simulink model "RailP_VD"  (R2018a)
settings: configuration reference "cs_ert" (kept outside this file)
values from neighbouring files (symbols this model uses):
  RailP_facFlt1PT1_C = 50.0    [RailP_VD.sldd]
  RailP_facFlt2PT1_C = 50.0    [RailP_VD.sldd]
  RailP_facFlt3PT1_C = 50.0    [RailP_VD.sldd]
  RailP_nDiffMax_C = 0.0    [RailP_VD.sldd]
  RailP_numMax_CUR : value not decoded    [RailP_VD.sldd]
  RailP_numMax_CURX : value not decoded    [RailP_VD.sldd]
  RailP_pFltWinNeg_CUR : value not decoded    [RailP_VD.sldd]
  RailP_pFltWinNeg_CURX : value not decoded    [RailP_VD.sldd]
  RailP_swtFlt_C = 1.0    [RailP_VD.sldd]
libraries: sllib x1
settings Model: DataDictionary=RailP_VD.sldd  Creator=zhoutinglin  LastModifiedBy=zhoutinglin

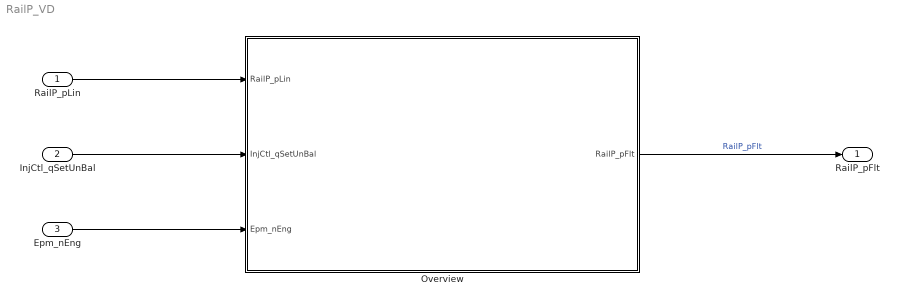
== system RailP_VD ==
  RailP_pLin : Inport  Description=Fuel pressure  OutMin=0  OutMax=2500  OutDataTypeStr=Press_bar1  Unit=bar  PortDimensions=[1 1]
  InjCtl_qSetUnBal : Inport  Description=Rail pressure setpoint  Port=2  OutMin=-319  OutMax=319  OutDataTypeStr=InjMass  Unit=bar  PortDimensions=[1 1]
  Epm_nEng : Inport  Description=Setpoint value (volume flow) of rail pressure governing  Port=3  OutMin=0  OutMax=6000  OutDataTypeStr=ERPM  Unit=mm^3/s  PortDimensions=[1 1]
  Overview : Subsystem
  RailP_pFlt : Outport
  wires:
  RailP_pLin/1 -> Overview/1(RailP_pLin)
  Epm_nEng/1 -> Overview/3(Epm_nEng)
  InjCtl_qSetUnBal/1 -> Overview/2(InjCtl_qSetUnBal)
  Overview/1(RailP_pFlt) -> RailP_pFlt/1  "RailP_pFlt"

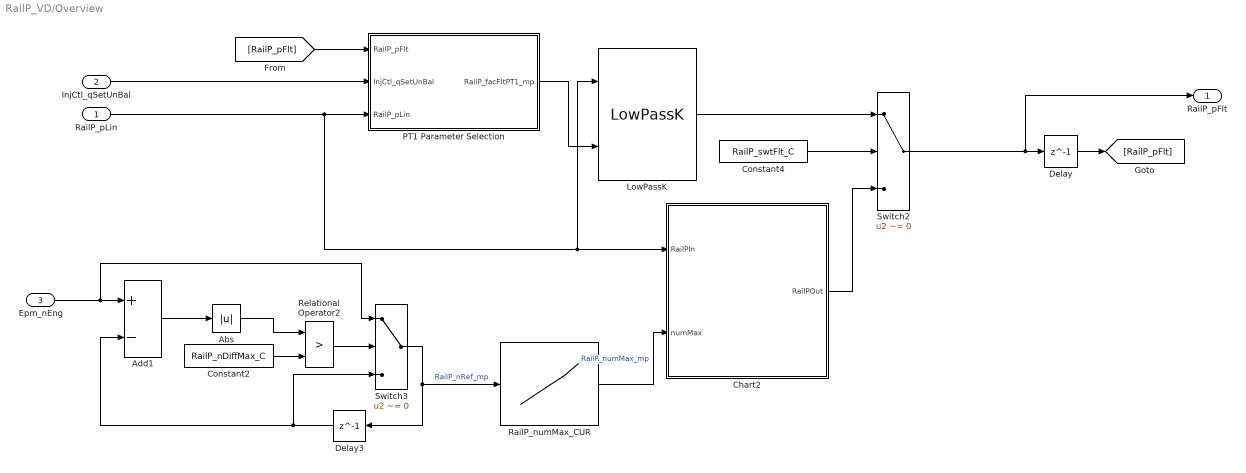
== system RailP_VD/Overview ==
  RailP_pLin : Inport  Tag=bar
  InjCtl_qSetUnBal : Inport  Tag=mg/hub  Port=2
  Epm_nEng : Inport  Port=3
  Abs : Abs
  Add1 : Sum  Inputs=+-  OutDataTypeStr=Inherit: Inherit via back propagation  RndMeth=Round  InputSameDT=on
  Chart2 : Stateflow chart  TreatAsAtomicUnit=on
  Constant2 : Constant  Value=RailP_nDiffMax_C
  Constant4 : Constant  Value=RailP_swtFlt_C
  Delay : Delay  DelayLength=1  InitialCondition=0
  Delay3 : Delay  DelayLength=1  InitialCondition=0
  LowPassK : sllib/LowPassK
      settings: SourceProductName=sllib
  PT1 Parameter Selection : Subsystem
  RailP_numMax_CUR : Lookup_n-D  NumberOfTableDimensions=1  BreakpointsForDimension1=RailP_numMax_CURX  IndexSearchMethod=Linear search  BeginIndexSearchUsingPreviousIndexResult=on  UseOneInputPortForAllInputData=on  Table=RailP_numMax_CUR  ExtrapMethod=Clip  UseLastTableValue=on  InternalRulePriority=Speed  OutDataTypeStr=Inherit: Inherit via back propagation  SaturateOnIntegerOverflow=on
  Relational Operator2 : RelationalOperator  Operator=>  OutDataTypeStr=boolean  RndMeth=Nearest  InputSameDT=on
  Switch2 : Switch  Criteria=u2 ~= 0  InputSameDT=on
  Switch3 : Switch  Criteria=u2 ~= 0  InputSameDT=on
  RailP_pFlt : Outport
  wires:
  Add1/1 -> Abs/1
  RailP_numMax_CUR/1 -> Chart2/2(numMax)  "RailP_numMax_mp"
  Delay/1 -> [RailP_pFlt]
  Delay3/1 -> Add1/2, Switch3/3
  Switch3/1 -> Delay3/1, RailP_numMax_CUR/1  "RailP_nRef_mp"
  Constant4/1 -> Switch2/2
  Constant2/1 -> Relational Operator2/2
  Chart2/1(RailPOut) -> Switch2/3
  Abs/1 -> Relational Operator2/1
  LowPassK/1 -> Switch2/1
  InjCtl_qSetUnBal/1 -> PT1 Parameter Selection/2(InjCtl_qSetUnBal)
  [RailP_pFlt] -> PT1 Parameter Selection/1(RailP_pFlt)
  Epm_nEng/1 -> Switch3/1, Add1/1
  Switch2/1 -> RailP_pFlt/1, Delay/1
  Relational Operator2/1 -> Switch3/2
  RailP_pLin/1 -> PT1 Parameter Selection/3(RailP_pLin), LowPassK/1, Chart2/1(RailPIn)
  PT1 Parameter Selection/1(RailP_facFltPT1_mp) -> LowPassK/2

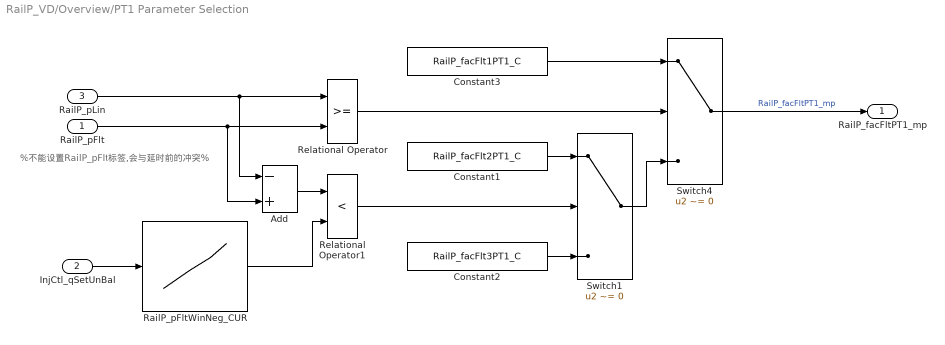
== system RailP_VD/Overview/PT1 Parameter Selection ==
  note: %不能设置RailP_pFlt标签,会与延时前的冲突%
  RailP_pFlt : Inport  Tag=mg/hub
  InjCtl_qSetUnBal : Inport  Tag=mg/hub  Port=2
  RailP_pLin : Inport  Tag=bar  Port=3
  Add : Sum  Inputs=-+  OutDataTypeStr=Inherit: Inherit via back propagation  InputSameDT=on
  Constant1 : Constant  Value=RailP_facFlt2PT1_C
  Constant2 : Constant  Value=RailP_facFlt3PT1_C
  Constant3 : Constant  Value=RailP_facFlt1PT1_C
  RailP_pFltWinNeg_CUR : Lookup_n-D  NumberOfTableDimensions=1  BreakpointsForDimension1=RailP_pFltWinNeg_CURX  IndexSearchMethod=Linear search  BeginIndexSearchUsingPreviousIndexResult=on  UseOneInputPortForAllInputData=on  Table=RailP_pFltWinNeg_CUR  ExtrapMethod=Clip  UseLastTableValue=on  InternalRulePriority=Speed  OutDataTypeStr=Inherit: Inherit via back propagation  SaturateOnIntegerOverflow=on
  Relational Operator : RelationalOperator  OutDataTypeStr=boolean  RndMeth=Nearest  InputSameDT=on
  Relational Operator1 : RelationalOperator  Operator=<  OutDataTypeStr=boolean  RndMeth=Nearest  InputSameDT=on
  Switch1 : Switch  Criteria=u2 ~= 0  InputSameDT=on
  Switch4 : Switch  Criteria=u2 ~= 0  InputSameDT=on
  RailP_facFltPT1_mp : Outport
  wires:
  Constant2/1 -> Switch1/3
  Constant1/1 -> Switch1/1
  InjCtl_qSetUnBal/1 -> RailP_pFltWinNeg_CUR/1
  RailP_pFltWinNeg_CUR/1 -> Relational Operator1/2
  Add/1 -> Relational Operator1/1
  Relational Operator1/1 -> Switch1/2
  Switch1/1 -> Switch4/3
  Switch4/1 -> RailP_facFltPT1_mp/1  "RailP_facFltPT1_mp"
  Constant3/1 -> Switch4/1
  Relational Operator/1 -> Switch4/2
  RailP_pFlt/1 -> Relational Operator/2, Add/2
  RailP_pLin/1 -> Relational Operator/1, Add/1

== stateflow chart RailP_VD/Overview/Chart2 ==
  (default) -> (junction 2) : {i=9;}
  (junction 2) -> (junction 5) [order 1] : [i>=1]
  (junction 5) -> (junction 7) : {RailPArray[i]=RailPArray[i-1];}
  (junction 7) -> (junction 2) : {i--;}
  (junction 2) -> (junction 1) [order 2] : {i=0;
      | RailPArray[0]=RailPIn;
      | RailPMax=RailPArray[0];}
  (junction 10) -> (junction 12) [order 1] : [RailPMax<RailPArray[i]]
  (junction 1) -> (junction 10) [order 1] : [i<numMax]
  (junction 10) -> (junction 16) [order 2]
  (junction 12) -> (junction 14) : {RailPMax=RailPArray[i];}
  (junction 16) -> (junction 1) : {i++;}
  (junction 1) -> (junction 20) [order 2] : {RailPOut=RailPMax;}
  (junction 14) -> (junction 16)
  data: RailPIn input; numMax input; RailPOut output; i local uint8; RailPMax local Press_bar1; RailPArray local Press_bar1 size=10
